simulink model "Statechart_Test_2_Ref1"  (R2016b)
settings: Solver=ode45  StartTime=0.0  StopTime=100  RelTol=1e-3  EnableMultiTasking=on
PreLoadFcn:
  | RED = 0;
  | ORANGE = 1;
  | GREEN = 2;
settings Model: Creator=The MathWorks, Inc.  LastModifiedBy=Rose
settings DataIOCC: LimitDataPoints=on  SaveFormat=Array  SaveOutput=off  SaveTime=off
settings OptimizationCC: ExpressionDepthLimit=2147483647  LifeSpan=1
settings DebuggingCC: UnderspecifiedInitializationDetection=Classic  MergeDetectMultiDrivingBlocksExec=none  FcnCallInpInsideContextMsg=warning  StateNameClashWarn=warning  SFUnexpectedBacktrackingDiag=warning  SFNoUnconditionalDefaultTransitionDiag=warning  SFExecutionAtInitializationDiag=none
settings HardwareCC: ProdBitPerPointer=32  ProdBitPerSizeT=32  ProdBitPerPtrDiffT=32  ProdLargestAtomicFloat=None  ProdIntDivRoundTo=Undefined  ProdEndianess=Unspecified  ProdWordSize=32  ProdHWDeviceType=32-bit Generic
settings ModelReferenceCC: PropagateSignalLabelsOutOfModel=off
settings RTWCC: SystemTargetFile=ert.tlc  TemplateMakefile=ert_default_tmf  Description=Embedded Coder
settings CodeAppCC: IgnoreCustomStorageClasses=off  CustomSymbolStrType=$N$R$M  InternalIdentifier=Classic
settings ERTTargetCC: GenerateSampleERTMain=on  ERTCustomFileTemplate=example_file_process.tlc  ConvertIfToSwitch=off  SuppressUnreachableDefaultCases=off
settings ConfigComp: CovMetricSettings=dw  CovHtmlReporting=on  CovSaveCumulativeToWorkspaceVar=on  CovSaveSingleToWorkspaceVar=on  CovExternalEMLEnable=off

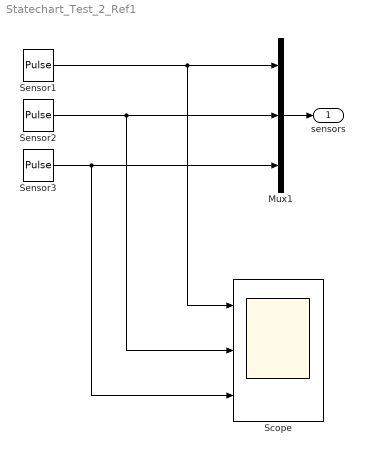
== system Statechart_Test_2_Ref1 ==
  Mux1 : Mux  Inputs=3
  Scope : Scope  NumInputPorts=3
  Sensor1 : DiscretePulseGenerator  PulseType=Time based  Amplitude=5  Period=5  PulseWidth=50  VectorParams1D=off
  Sensor2 : DiscretePulseGenerator  PulseType=Time based  Amplitude=5  Period=5  PulseWidth=80  VectorParams1D=off
  Sensor3 : DiscretePulseGenerator  PulseType=Time based  Amplitude=5  Period=5  PulseWidth=50  VectorParams1D=off
  sensors : Outport  OutDataTypeStr=double  PortDimensions=3
  wires:
  Mux1/1 -> sensors/1
  Sensor1/1 -> Mux1/1, Scope/1
  Sensor2/1 -> Mux1/2, Scope/2
  Sensor3/1 -> Scope/3, Mux1/3
